simulink model "Look"  (R2018b)
settings: Solver=VariableStepAuto  StartTime=0.0  StopTime=10.0  RelTol=1e-3
settings Model: Creator=kekos  LastModifiedBy=kekos

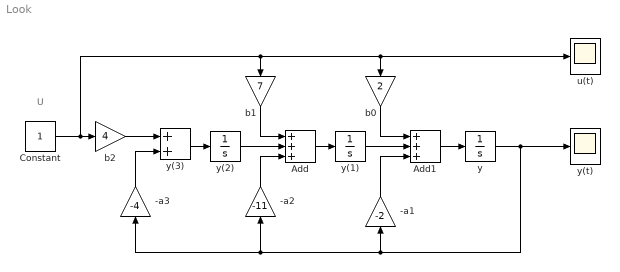
== system Look ==
  note: U
  -a1 : Gain  Gain=-2
  -a2 : Gain  Gain=-11
  -a3 : Gain  Gain=-4
  Add : Sum  Inputs=3
  Add1 : Sum  Inputs=3
  Constant : Constant
  b0 : Gain  Gain=2
  b1 : Gain  Gain=7
  b2 : Gain  Gain=4
  u(t) : Scope
  y : Integrator  InitialCondition=1
  y(1) : Integrator  InitialCondition=0.3
  y(2) : Integrator  InitialCondition=3.4
  y(3) : Sum  Inputs=2
  y(t) : Scope
  wires:
  y(3)/1 -> y(2)/1
  b2/1 -> y(3)/1
  b1/1 -> Add/1
  y(2)/1 -> Add/2
  Add/1 -> y(1)/1
  Add1/1 -> y/1
  b0/1 -> Add1/1
  y(1)/1 -> Add1/2
  y/1 -> y(t)/1, -a3/1, -a2/1, -a1/1
  -a3/1 -> y(3)/2
  -a2/1 -> Add/3
  -a1/1 -> Add1/3
  Constant/1 -> u(t)/1, b0/1, b1/1, b2/1
